simulink model "BRGH_MRC_simulink"  (R2023b)
settings: Solver=VariableStepAuto  StartTime=0.0  StopTime=simTime  RelTol=1e-3
values from neighbouring files (symbols this model uses):
  freq = .5    (= 0.5)    [MRC_script.m]
  kp = b1    (= 0.3)    [MRC_script.m]
  Lambda0 = [1 lambda0]    [MRC_script.m]
  r = 1    [MRC_script.m]
  Rm = [1 0.1]    [MRC_script.m]
  Rp = [1 a1 a0]    [MRC_script.m]
  Zm = 1    [MRC_script.m]
  Zp = [0 1 b0/b1]    [MRC_script.m]
settings Model: Creator=eliasoa  LastModifiedBy=eliasoa

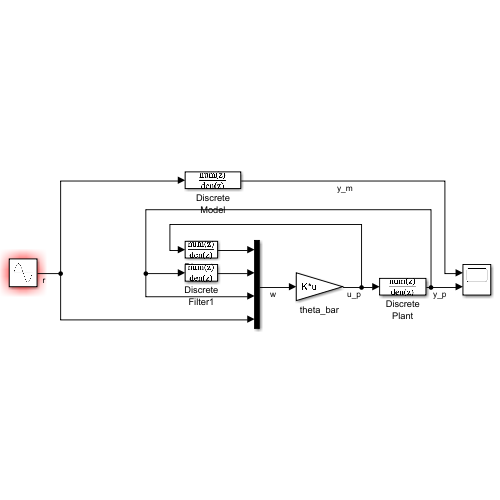
[thumbnail: Simulink's stored preview of the top-level diagram]
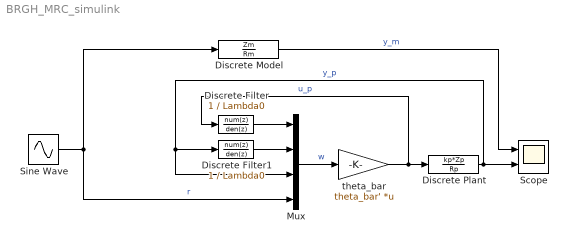
== system BRGH_MRC_simulink ==
  Discrete Filter : DiscreteTransferFcn  Numerator=1  Denominator=Lambda0
  Discrete Filter1 : DiscreteTransferFcn  Numerator=1  Denominator=Lambda0
  Discrete Model : DiscreteTransferFcn  Numerator=Zm  Denominator=Rm
  Discrete Plant : DiscreteTransferFcn  Numerator=kp*Zp  Denominator=Rp
  Mux : Mux
  Scope : Scope  NumInputPorts=2
  Sine Wave : Sin  Amplitude=r  Frequency=freq  SampleTime=0
  theta_bar : Gain  Gain=theta_bar'  Multiplication=Matrix(K*u)
  wires:
  Discrete Model/1 -> Scope/1  "y_m"
  Sine Wave/1 -> Discrete Model/1, Mux/4  "r"
  Mux/1 -> theta_bar/1  "w"
  Discrete Plant/1 -> Scope/2, Discrete Filter1/1, Mux/3  "y_p"
  theta_bar/1 -> Discrete Plant/1, Discrete Filter/1  "u_p"
  Discrete Filter1/1 -> Mux/2
  Discrete Filter/1 -> Mux/1
